simulink model "A3_1_VorKin_testing"  (R2023a)
settings: Solver=VariableStepAuto  StartTime=0.0  StopTime=10.0  RelTol=1e-3
values from neighbouring files (symbols this model uses):
  params = [l2 l3]    [A3_1_init_VorKin.m]    (also in A3_2_init_InvKin.m; init_InvKin.m)
settings Model: Creator=Flo  LastModifiedBy=Flo

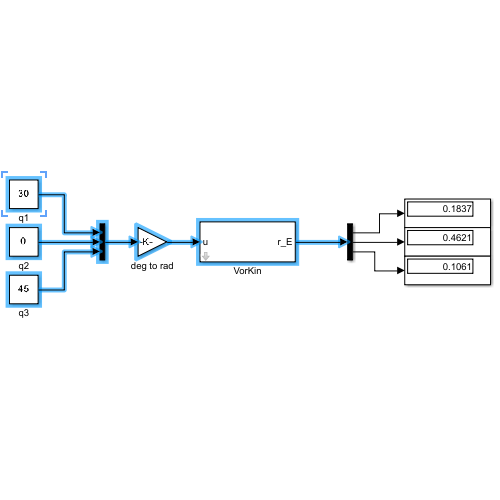
[thumbnail: Simulink's stored preview of the top-level diagram]
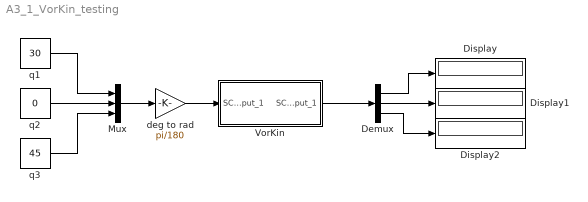
== system A3_1_VorKin_testing ==
  Demux : Demux  Outputs=3
  Display : Display
  Display1 : Display
  Display2 : Display
  Mux : Mux  Inputs=3
  VorKin : Subsystem  mask{SC_param_0=params}
      mask prompts: SC_param_0 "params"
      mask Display:
      | port_label('input', 1, 'u');
      | port_label('output', 1, 'r_E');
  deg to rad : Gain  Gain=pi/180
  q1 : Constant  Value=30
  q2 : Constant  Value=0
  q3 : Constant  Value=45
  wires:
  q2/1 -> Mux/2
  q3/1 -> Mux/3
  q1/1 -> Mux/1
  Mux/1 -> deg to rad/1
  deg to rad/1 -> VorKin/1(SC_input_1)
  VorKin/1(SC_output_1) -> Demux/1
  Demux/3 -> Display2/1
  Demux/2 -> Display1/1
  Demux/1 -> Display/1

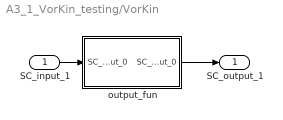
== system A3_1_VorKin_testing/VorKin ==
  SC_input_1 : Inport
  output_fun : MATLAB Function  TreatAsAtomicUnit=on
  SC_output_1 : Outport
  wires:
  SC_input_1/1 -> output_fun/1(SC_input_0)
  output_fun/1(SC_output_0) -> SC_output_1/1

== matlab function A3_1_VorKin_testing/VorKin/output_fun ==
  data: SC_input_0 input size=[3]; SC_output_0 output size=[3]; SC_param_0 parameter size=[2]
function SC_output_0  = y_fun(SC_input_0, SC_param_0)
    SC_output_0 = zeros(3,1);
    t1 = SC_input_0(1);
    t2 = cos(t1);
    t3 = SC_input_0(3);
    t4 = cos(t3);
    t5 = SC_param_0(2);
    t7 = SC_input_0(2);
    t8 = sin(t7);
    t9 = SC_param_0(1);
    t11 = t4 * t5 + t8 * t9;
    SC_output_0(1) = t11 * t2;
    t12 = sin(t3);
    t14 = cos(t7);
    SC_output_0(2) = t12 * t5 + t14 * t9;
    t16 = sin(t1);
    SC_output_0(3) = t16 * t11;
end
